simulink model "traj_test_adept_18"  (R2013b)
settings: Solver=ode4  StartTime=0.0  StopTime=2.18  FixedStep=0.001  RelTol=1e-3
settings Model: Creator=lucius  LastModifiedBy=lucius
settings DataIOCC: LimitDataPoints=off

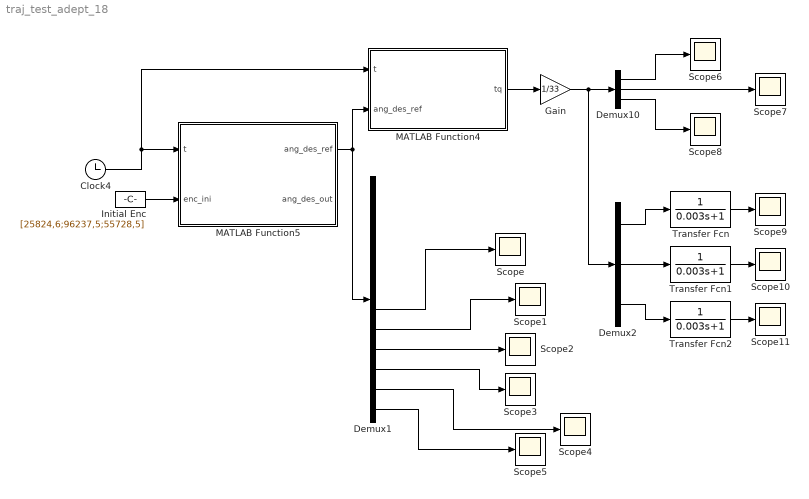
== system traj_test_adept_18 ==
  Clock4 : Clock
  Demux1 : Demux  Outputs=12
  Demux10 : Demux  Outputs=3
  Demux2 : Demux  Outputs=3
  Gain : Gain  Gain=1/33
  Initial Enc : Constant  Value=[25824,6;96237,5;55728,5]
  MATLAB Function4 : MATLAB Function  TreatAsAtomicUnit=on
  MATLAB Function5 : MATLAB Function  TreatAsAtomicUnit=on
  Scope{,1..11} (12 alike) : Scope
      Scope10 settings: SaveName=ScopeData9
      Scope11 settings: SaveName=ScopeData10
      Scope2 settings: SaveName=ScopeData2
      Scope3 settings: SaveName=ScopeData3
      Scope4 settings: SaveName=ScopeData4
      Scope5 settings: SaveName=ScopeData5
      Scope6 settings: SaveName=ScopeData6
      Scope7 settings: SaveName=ScopeData7
      Scope8 settings: SaveName=ScopeData8
      Scope9 settings: SaveName=ScopeData11
  Transfer Fcn : TransferFcn  Denominator=[0.003 1]
  Transfer Fcn1 : TransferFcn  Denominator=[0.003 1]
  Transfer Fcn2 : TransferFcn  Denominator=[0.003 1]
  wires:
  Initial Enc/1 -> MATLAB Function5/2(enc_ini)
  MATLAB Function5/1(ang_des_ref) -> MATLAB Function4/2(ang_des_ref), Demux1/1
  Demux10/1 -> Scope6/1
  Demux10/2 -> Scope7/1
  Demux10/3 -> Scope8/1
  MATLAB Function4/1(tq) -> Gain/1
  Demux1/12 -> Scope5/1
  Demux1/11 -> Scope4/1
  Demux1/10 -> Scope3/1
  Demux1/7 -> Scope/1
  Demux1/8 -> Scope1/1
  Demux1/9 -> Scope2/1
  Clock4/1 -> MATLAB Function4/1(t), MATLAB Function5/1(t)
  Gain/1 -> Demux2/1, Demux10/1
  Transfer Fcn/1 -> Scope9/1
  Demux2/1 -> Transfer Fcn/1
  Demux2/2 -> Transfer Fcn1/1
  Transfer Fcn1/1 -> Scope10/1
  Demux2/3 -> Transfer Fcn2/1
  Transfer Fcn2/1 -> Scope11/1

== matlab function traj_test_adept_18/MATLAB Function4 ==
  data: t input; tq output; ang_des_ref input
function tq = ctf(t,ang_des_ref)
T=2;
if t<T
    tq=[0;0;0];
else
    torq=dltsdy([ang_des_ref(1);ang_des_ref(2);ang_des_ref(3)],[ang_des_ref(4);ang_des_ref(5);ang_des_ref(6)],[ang_des_ref(7);ang_des_ref(8);ang_des_ref(9)],[ang_des_ref(10);ang_des_ref(11);ang_des_ref(12)]);
    tq=-[torq(1);torq(3);torq(2)];%convert to the real torq comand
end

== matlab function traj_test_adept_18/MATLAB Function5 ==
  data: ang_des_ref output; t input; enc_ini input; ang_des_out output
function [ang_des_ref,ang_des_out] = traj_adept(t,enc_ini)
% /***********************************************************************
% * Name:       Adept Motion Trajectory of Delta Robot
% * Type:       Embedded Matlab Function
% * Author:     Yujiong Liu
% * Date:       2015.6.9
% * 
% * Input:      enc_ini     Initial absolute encoder value
% *             t           Simulation time
% * 
% * Output:     ang_des     Desire joint angle
% *             ang_des_ref Desire joint angle reference, 1-3 ang_dd, 4-6
% *                         x_dd
% * Function:   As shown in Name 
% ***********************************************************************/

%***********************REFERENCE****************************************
%LIMIT&ABSOLUTE NUMBER
%Axis#      Limit   Absolute Position
%1          -45     14circles   +1784
%           100     0circles    +98713

%2          -45     13circles   +120485
%           100     0circles    +87782

%3          -45     13circles   +77696
%           100     0circles    +44275
%********************Time to execute the p2p motion***********************
T=2;
%****************************COMPUTATION**********************************
if t<T
%1 Move to the start point of the adept motion in T
%convert initial encoder value to joint angle
ang_ini=[0,0,0];
%Axis#1
ang_ini(1)=(131072*enc_ini(1,2)+enc_ini(1,1)-98713)*pi*29/36/(14*131072+1784-98713)-5*pi/9;
%Axis#2
ang_ini(2)=(131072*enc_ini(2,2)+enc_ini(2,1)-87782)*pi*29/36/(13*131072+120485-87782)-5*pi/9;
%Axis#3
ang_ini(3)=(131072*enc_ini(3,2)+enc_ini(3,1)-44275)*pi*29/36/(13*131072+77696-44275)-5*pi/9;

%the joint angle of the adept motion start point[0,-0.15,0.67777]
%convert the kinematics angle to real angle
ang_end=-[0.061087346682504,-0.243715535550272,0.345186315942479];

%trajectory in joint space
ang_des_out=[0,0,0];
ang_des_out(1)=(2*(ang_ini(1)-ang_end(1))/(T^3))*t^3+(3*(ang_end(1)-ang_ini(1))/(T^2))*t^2+ang_ini(1);
ang_des_out(2)=(2*(ang_ini(2)-ang_end(2))/(T^3))*t^3+(3*(ang_end(2)-ang_ini(2))/(T^2))*t^2+ang_ini(2);
ang_des_out(3)=(2*(ang_ini(3)-ang_end(3))/(T^3))*t^3+(3*(ang_end(3)-ang_ini(3))/(T^2))*t^2+ang_ini(3);
ang_des=-[ang_des_out(1);ang_des_out(3);ang_des_out(2)];

ang_des_d=[0,0,0];
ang_des_d(1)=-((2*(ang_ini(1)-ang_end(1))/(T^3))*(3*t^2)+(3*(ang_end(1)-ang_ini(1))/(T^2))*(2*t));
ang_des_d(2)=-((2*(ang_ini(3)-ang_end(3))/(T^3))*(3*t^2)+(3*(ang_end(3)-ang_ini(3))/(T^2))*(2*t));
ang_des_d(3)=-((2*(ang_ini(2)-ang_end(2))/(T^3))*(3*t^2)+(3*(ang_end(2)-ang_ini(2))/(T^2))*(2*t));

ang_des_dd=[0,0,0];
ang_des_dd(1)=-((2*(ang_ini(1)-ang_end(1))/(T^3))*(6*t)+(3*(ang_end(1)-ang_ini(1))/(T^2))*2);
ang_des_dd(2)=-((2*(ang_ini(3)-ang_end(3))/(T^3))*(6*t)+(3*(ang_end(3)-ang_ini(3))/(T^2))*2);
ang_des_dd(3)=-((2*(ang_ini(2)-ang_end(2))/(T^3))*(6*t)+(3*(ang_end(2)-ang_ini(2))/(T^2))*2);

ps_t_dd=dltacc(ang_des,ang_des_d,ang_des_dd);
ang_des_ref=[ang_des(1),ang_des(2),ang_des(3),ang_des_d(1),ang_des_d(2),ang_des_d(3),ang_des_dd(1),ang_des_dd(2),ang_des_dd(3),ps_t_dd(1),ps_t_dd(2),ps_t_dd(3)];
%2 Execute the adept motion
else
    %*******************************Path Parameter****************************
%             C********************************D          
%        *                                         *
%      *                      |Z                       *
%    B*                       |                         *E
%    A*                       |________Y                *F
X_A=[0,-0.15,0.677772085586298];
X_B=[0,-0.15,0.667772085586298];
X_C=[0,-0.135,0.652772085586298];
X_D=[0,0.135,0.652772085586298];
X_E=[0,0.15,0.667772085586298];
X_F=[0,0.15,0.677772085586298];
V_A=0;
V_B=0.94;%%%%
V_C=1.2;%%%%
V_D=1.1;%%%%
V_E=0.85;%%%%
V_F=0;
T_AB=0.016;%%%%
T_BC=0.021;%%%%
T_CD=0.102;%%%%
T_DE=0.024;%%%%
T_EF=0.017;%%%%
%********************Auxiliary Parameter*********************************
%Circle#1
Cen_C1=[0,-0.135,0.667772085586298];             %Center
Nor_C1=[-1,0,0];            %Normal vector of circle plane, left hand rule
Theta_C1=pi/2;              %Rotation angle
Rad_C1=0.015;               %Radius of circle
%Circle#2
Cen_C2=[0,0.135,0.667772085586298];             %Center
Nor_C2=[-1,0,0];             %Normal vector of circle plane, left hand rule
Theta_C2=pi/2;              %Rotation angle
Rad_C2=0.015;               %Radius of circle
    if t<T_AB+T                    %segment AB LINE
        Vec_AB=X_B-X_A;
        l_AB=norm(Vec_AB);
        V_A=V_A/l_AB;
        V_B=V_B/l_AB;
        k_AB=(V_A+V_B-2/T_AB)*((t-T)^3)/(T_AB^2)+(3/T_AB-2*V_A-V_B)*((t-T)^2)/T_AB+V_A*(t-T);
        ps_t=X_A+k_AB*Vec_AB;
        ang_des=dltgik(ps_t)';
        ang_des_out=-[ang_des(1),ang_des(3),ang_des(2)];
        %for ang_des_ref
        k_AB_d=(V_A+V_B-2/T_AB)*(3*(t-T)^2)/(T_AB^2)+(3/T_AB-2*V_A-V_B)*(2*(t-T))/T_AB+V_A;
        k_AB_dd=(V_A+V_B-2/T_AB)*6*(t-T)/(T_AB^2)+(3/T_AB-2*V_A-V_B)*2/T_AB;
        ps_t_d=k_AB_d*Vec_AB;
        ps_t_dd=k_AB_dd*Vec_AB;
        ang_des_dd=dltinvacc(ang_des,ps_t,ps_t_d,ps_t_dd);
        ang_des_d=dltinvjc([ps_t(1);ps_t(2);ps_t(3)])*[ps_t_d(1);ps_t_d(2);ps_t_d(3)];
        ang_des_ref=[ang_des(1),ang_des(2),ang_des(3),ang_des_d(1),ang_des_d(2),ang_des_d(3),ang_des_dd(1),ang_des_dd(2),ang_des_dd(3),ps_t_dd(1),ps_t_dd(2),ps_t_dd(3)];
      else if t<T_AB+T_BC+T           %segment BC CIRCLE
              theta_BC=(V_B+V_C-2*Rad_C1*Theta_C1/T_BC)*((t-T_AB-T)^3)/(Rad_C1*T_BC^2)+(3*Rad_C1*Theta_C1/T_BC-2*V_B-V_C)*((t-T_AB-T)^2)/(Rad_C1*T_BC)+V_B*(t-T_AB-T)/Rad_C1;
              temp_C1=cross(X_B-Cen_C1,Nor_C1);
              ens_temp_C1=temp_C1/norm(temp_C1);
              p_dp_C1=Rad_C1*sin(theta_BC)*ens_temp_C1;
              ps_t=Cen_C1+cos(theta_BC)*(X_B-Cen_C1)+p_dp_C1;
              ang_des=dltgik(ps_t)';
              ang_des_out=-[ang_des(1),ang_des(3),ang_des(2)];
              %for ang_des_ref
              theta_BC_d=(V_B+V_C-2*Rad_C1*Theta_C1/T_BC)*(3*(t-T_AB-T)^2)/(Rad_C1*T_BC^2)+(3*Rad_C1*Theta_C1/T_BC-2*V_B-V_C)*(2*(t-T_AB-T))/(Rad_C1*T_BC)+V_B/Rad_C1;
              theta_BC_dd=(V_B+V_C-2*Rad_C1*Theta_C1/T_BC)*(6*(t-T_AB-T))/(Rad_C1*T_BC^2)+(3*Rad_C1*Theta_C1/T_BC-2*V_B-V_C)*2/(Rad_C1*T_BC);
              ps_t_d=-theta_BC_d*sin(theta_BC)*(X_B-Cen_C1)+theta_BC_d*cos(theta_BC)*Rad_C1*ens_temp_C1;
              ps_t_dd=-(theta_BC_d^2*cos(theta_BC)+theta_BC_dd*sin(theta_BC))*(X_B-Cen_C1)+(theta_BC_dd*cos(theta_BC)-theta_BC_d^2*sin(theta_BC))*Rad_C1*ens_temp_C1;
%               ops_t=ps_t-Cen_C1;
%               temp_1_C1=cross(ops_t,Nor_C1);
%               ens_temp_1_C1=temp_1_C1/norm(temp_1_C1);
%               ps_t_d=theta_BC_d*ens_temp_1_C1;
%               ps_t_dd=theta_BC_dd*ens_temp_1_C1;
              ang_des_dd=dltinvacc(ang_des,ps_t,ps_t_d,ps_t_dd);
              ang_des_d=dltinvjc([ps_t(1);ps_t(2);ps_t(3)])*[ps_t_d(1);ps_t_d(2);ps_t_d(3)];
              ang_des_ref=[ang_des(1),ang_des(2),ang_des(3),ang_des_d(1),ang_des_d(2),ang_des_d(3),ang_des_dd(1),ang_des_dd(2),ang_des_dd(3),ps_t_dd(1),ps_t_dd(2),ps_t_dd(3)];
            else if t<T_AB+T_BC+T_CD+T                      %segment CD LINE
                    Vec_CD=X_D-X_C;
                    l_CD=norm(Vec_CD);
                    V_C=V_C/l_CD;
                    V_D=V_D/l_CD;
                    k_CD=(V_C+V_D-2/T_CD)*((t-T_AB-T_BC-T)^3)/(T_CD^2)+(3/T_CD-2*V_C-V_D)*((t-T_AB-T_BC-T)^2)/T_CD+V_C*(t-T_AB-T_BC-T);
                    ps_t=X_C+k_CD*Vec_CD;
                    ang_des=dltgik(ps_t)';
                    ang_des_out=-[ang_des(1),ang_des(3),ang_des(2)];
                    %for ang_des_ref
                    k_CD_d=(V_C+V_D-2/T_CD)*(3*(t-T_AB-T_BC-T)^2)/(T_CD^2)+(3/T_CD-2*V_C-V_D)*(2*(t-T_AB-T_BC-T))/T_CD+V_C;
                    k_CD_dd=(V_C+V_D-2/T_CD)*(6*(t-T_AB-T_BC-T))/(T_CD^2)+(3/T_CD-2*V_C-V_D)*2/T_CD;
                    ps_t_d=k_CD_d*Vec_CD;
                    ps_t_dd=k_CD_dd*Vec_CD;
                    ang_des_dd=dltinvacc(ang_des,ps_t,ps_t_d,ps_t_dd);
                    ang_des_d=dltinvjc([ps_t(1);ps_t(2);ps_t(3)])*[ps_t_d(1);ps_t_d(2);ps_t_d(3)];
                    ang_des_ref=[ang_des(1),ang_des(2),ang_des(3),ang_des_d(1),ang_des_d(2),ang_des_d(3),ang_des_dd(1),ang_des_dd(2),ang_des_dd(3),ps_t_dd(1),ps_t_dd(2),ps_t_dd(3)];
                  else if t<T_AB+T_BC+T_CD+T_DE+T             %segment DE CIRCLE
                          theta_DE=(V_D+V_E-2*Rad_C2*Theta_C2/T_DE)*((t-T_AB-T_BC-T_CD-T)^3)/(Rad_C2*T_DE^2)+(3*Rad_C2*Theta_C2/T_DE-2*V_D-V_E)*((t-T_AB-T_BC-T_CD-T)^2)/(Rad_C2*T_DE)+V_D*(t-T_AB-T_BC-T_CD-T)/Rad_C2;
                          temp_C2=cross(X_D-Cen_C2,Nor_C2);
                          ens_temp_C2=temp_C2/norm(temp_C2);
                           p_dp_C2=Rad_C2*sin(theta_DE)*ens_temp_C2;
                           ps_t=Cen_C2+cos(theta_DE)*(X_D-Cen_C2)+p_dp_C2;
                           ang_des=dltgik(ps_t)';
                           ang_des_out=-[ang_des(1),ang_des(3),ang_des(2)];
                           %for ang_des_ref
                           theta_DE_d=(V_D+V_E-2*Rad_C2*Theta_C2/T_DE)*(3*(t-T_AB-T_BC-T_CD-T)^2)/(Rad_C2*T_DE^2)+(3*Rad_C2*Theta_C2/T_DE-2*V_D-V_E)*(2*(t-T_AB-T_BC-T_CD-T))/(Rad_C2*T_DE)+V_D/Rad_C2;
                           theta_DE_dd=(V_D+V_E-2*Rad_C2*Theta_C2/T_DE)*(6*(t-T_AB-T_BC-T_CD-T))/(Rad_C2*T_DE^2)+(3*Rad_C2*Theta_C2/T_DE-2*V_D-V_E)*2/(Rad_C2*T_DE);
                           ps_t_d=-theta_DE_d*sin(theta_DE)*(X_D-Cen_C2)+theta_DE_d*cos(theta_DE)*Rad_C2*ens_temp_C2;
                           ps_t_dd=-(theta_DE_d^2*cos(theta_DE)+theta_DE_dd*sin(theta_DE))*(X_D-Cen_C2)+(theta_DE_dd*cos(theta_DE)-theta_DE_d^2*sin(theta_DE))*Rad_C2*ens_temp_C2;
%                            ops_t=ps_t-Cen_C2;
%                            temp_1_C2=cross(ops_t,Nor_C2);
%                            ens_temp_1_C2=temp_1_C2/norm(temp_1_C2);
%                            ps_t_d=theta_DE_d*ens_temp_1_C2;
%                            ps_t_dd=theta_DE_dd*ens_temp_1_C2;
                           ang_des_dd=dltinvacc(ang_des,ps_t,ps_t_d,ps_t_dd);
                           ang_des_d=dltinvjc([ps_t(1);ps_t(2);ps_t(3)])*[ps_t_d(1);ps_t_d(2);ps_t_d(3)];
                           ang_des_ref=[ang_des(1),ang_des(2),ang_des(3),ang_des_d(1),ang_des_d(2),ang_des_d(3),ang_des_dd(1),ang_des_dd(2),ang_des_dd(3),ps_t_dd(1),ps_t_dd(2),ps_t_dd(3)];
                       else if t<T_AB+T_BC+T_CD+T_DE+T_EF+T    %segment EF LINE
                               Vec_EF=X_F-X_E;
                               l_EF=norm(Vec_EF);
                               V_E=V_E/l_EF;
                               V_F=V_F/l_EF;
                               k_EF=(V_E+V_F-2/T_EF)*((t-T_AB-T_BC-T_CD-T_DE-T)^3)/(T_EF^2)+(3/T_EF-2*V_E-V_F)*((t-T_AB-T_BC-T_CD-T_DE-T)^2)/T_EF+V_E*(t-T_AB-T_BC-T_CD-T_DE-T);
                               ps_t=X_E+k_EF*Vec_EF;
                               ang_des=dltgik(ps_t)';
                               ang_des_out=-[ang_des(1),ang_des(3),ang_des(2)];
                               %for ang_des_ref
                               k_EF_d=(V_E+V_F-2/T_EF)*(3*(t-T_AB-T_BC-T_CD-T_DE-T)^2)/(T_EF^2)+(3/T_EF-2*V_E-V_F)*(2*(t-T_AB-T_BC-T_CD-T_DE-T))/T_EF+V_E;
                               k_EF_dd=(V_E+V_F-2/T_EF)*(6*(t-T_AB-T_BC-T_CD-T_DE-T))/(T_EF^2)+(3/T_EF-2*V_E-V_F)*2/T_EF;
                               ps_t_d=k_EF_d*Vec_EF;
                               ps_t_dd=k_EF_dd*Vec_EF;
                               ang_des_dd=dltinvacc(ang_des,ps_t,ps_t_d,ps_t_dd);
                               ang_des_d=dltinvjc([ps_t(1);ps_t(2);ps_t(3)])*[ps_t_d(1);ps_t_d(2);ps_t_d(3)];
                               ang_des_ref=[ang_des(1),ang_des(2),ang_des(3),ang_des_d(1),ang_des_d(2),ang_des_d(3),ang_des_dd(1),ang_des_dd(2),ang_des_dd(3),ps_t_dd(1),ps_t_dd(2),ps_t_dd(3)];
                            else ps_t=X_F;                   %wait to terminate
                                ang_des=dltgik(ps_t)';
                                ang_des_out=-[ang_des(1),ang_des(3),ang_des(2)];
                                ang_des_ref=[0,0,0,0,0,0,0,0,0,0,0,0];
                            end
                       end
                  end
            end
    end
end
